simulink model "controlador2"  (R2019a)
settings: Solver=FixedStepDiscrete  StartTime=0.0  StopTime=150  FixedStep=0.1  RelTol=1e-3
undefined symbols (not defined in the file): Angular, Linear
libraries: robotlib x11, fuzblock x1, robotcorelib x1
settings Model: EnablePacing=on  Creator=pizarro  LastModifiedBy=Álvaro Zamorano

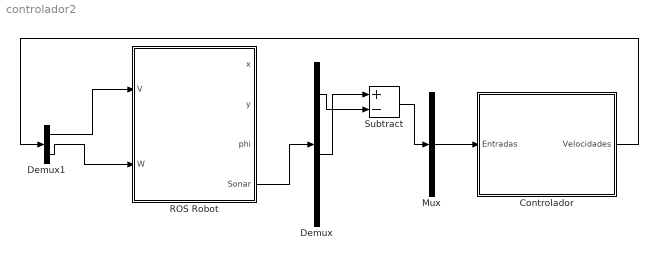
== system controlador2 ==
  Controlador : Subsystem
  Demux : Demux  Outputs=8
  Demux1 : Demux  Outputs=2
  Mux : Mux  Inputs=1
  ROS Robot : Subsystem
  Subtract : Sum  Inputs=+-
  wires:
  ROS Robot/4(Sonar) -> Demux/1
  Mux/1 -> Controlador/1(Entradas)
  Demux1/1 -> ROS Robot/1(V)
  Demux1/2 -> ROS Robot/2(W)
  Controlador/1(Velocidades) -> Demux1/1
  Demux/5 -> Subtract/1
  Subtract/1 -> Mux/1
  Demux/2 -> Subtract/2

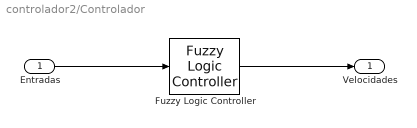
== system controlador2/Controlador ==
  Entradas : Inport
  Fuzzy Logic Controller : fuzblock/Fuzzy Logic  Controller  FIS='Controlador2.fis'  OutputSampleNumber=101  DataType=double  FuzzifiedInputs=off  RuleFiringStrengths=off  RuleOutputs=off  AggregatedOutputs=off  SimulateUsing=Interpreted execution  OutOfRangeInputValueMessage=warning  NoRuleFiredMessage=warning  EmptyOutputFuzzySetMessage=warning
  Velocidades : Outport
  wires:
  Fuzzy Logic Controller/1 -> Velocidades/1
  Entradas/1 -> Fuzzy Logic Controller/1

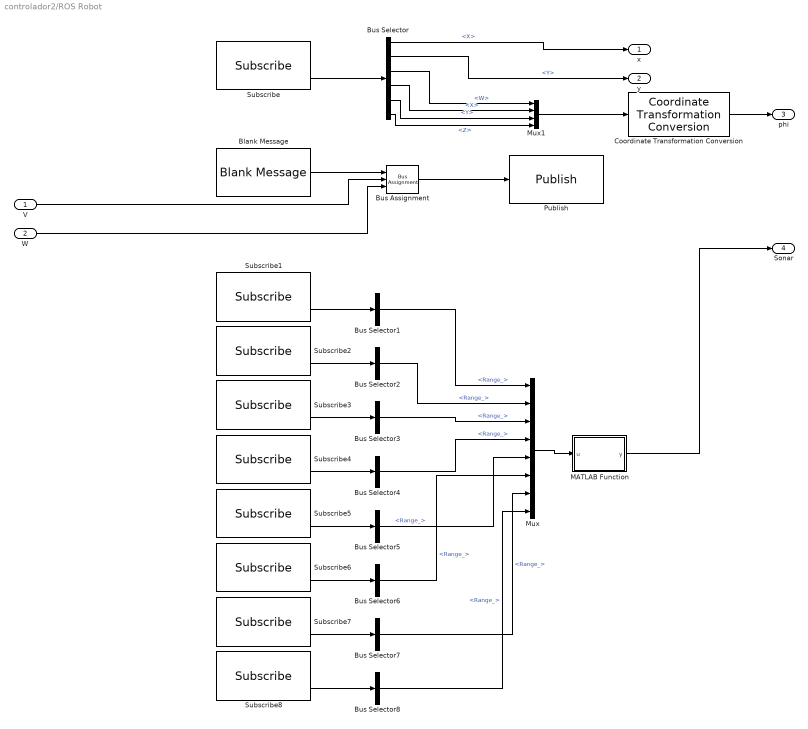
== system controlador2/ROS Robot ==
  V : Inport
  W : Inport  Port=2
  Blank Message : robotlib/Blank Message  messageClass=Message  entityType=geometry_msgs/Twist  messageType=geometry_msgs/Twist  SampleTime=-1
      settings: SourceProductBaseCode=RO
  Bus Assignment : BusAssignment  AssignedSignals=Linear.X,Angular.Z
  Bus Selector : BusSelector  OutputSignals=Pose.Pose.Position.X,Pose.Pose.Position.Y,Pose.Pose.Orientation.W,Pose.Pose.Orientation.X,Pose.Pose.Orientation.Y,Pose.Pose.Orientation.Z
  Bus Selector{1..8} (8 alike) : BusSelector  OutputSignals=Range_
  Coordinate Transformation Conversion : robotcorelib/Coordinate Transformation Conversion  InputRepresentation=Quaternion  InputEulerSequence=ZYX  ShowTrVecInputPort=on  OutputRepresentation=Euler Angles  OutputEulerSequence=ZYX  ShowTrVecOutputPort=on  SimulateUsing=Interpreted execution
      settings: SourceProductBaseCode=RO
  MATLAB Function : MATLAB Function  TreatAsAtomicUnit=on
  Mux : Mux  Inputs=8
  Mux1 : Mux
  Publish : robotlib/Publish  topicSource=Select from ROS network  topic=/robot0/cmd_vel  messageType=geometry_msgs/Twist  messageQueueLength=1
      settings: SourceProductBaseCode=RO
  Subscribe : robotlib/Subscribe  topicSource=Specify your own  topic=/robot0/odom  messageType=nav_msgs/Odometry  sampleTime=-1  messageQueueLength=1
      settings: SourceProductBaseCode=RO
  Subscribe1 : robotlib/Subscribe  topicSource=Select from ROS network  topic=/robot0/sonar_0  messageType=sensor_msgs/Range  sampleTime=-1  messageQueueLength=1
      settings: SourceProductBaseCode=RO
  Subscribe2 : robotlib/Subscribe  topicSource=Select from ROS network  topic=/robot0/sonar_1  messageType=sensor_msgs/Range  sampleTime=-1  messageQueueLength=1
      settings: SourceProductBaseCode=RO
  Subscribe3 : robotlib/Subscribe  topicSource=Select from ROS network  topic=/robot0/sonar_2  messageType=sensor_msgs/Range  sampleTime=-1  messageQueueLength=1
      settings: SourceProductBaseCode=RO
  Subscribe4 : robotlib/Subscribe  topicSource=Select from ROS network  topic=/robot0/sonar_3  messageType=sensor_msgs/Range  sampleTime=-1  messageQueueLength=1
      settings: SourceProductBaseCode=RO
  Subscribe5 : robotlib/Subscribe  topicSource=Select from ROS network  topic=/robot0/sonar_4  messageType=sensor_msgs/Range  sampleTime=-1  messageQueueLength=1
      settings: SourceProductBaseCode=RO
  Subscribe6 : robotlib/Subscribe  topicSource=Select from ROS network  topic=/robot0/sonar_5  messageType=sensor_msgs/Range  sampleTime=-1  messageQueueLength=1
      settings: SourceProductBaseCode=RO
  Subscribe7 : robotlib/Subscribe  topicSource=Select from ROS network  topic=/robot0/sonar_6  messageType=sensor_msgs/Range  sampleTime=-1  messageQueueLength=1
      settings: SourceProductBaseCode=RO
  Subscribe8 : robotlib/Subscribe  topicSource=Select from ROS network  topic=/robot0/sonar_7  messageType=sensor_msgs/Range  sampleTime=-1  messageQueueLength=1
      settings: SourceProductBaseCode=RO
  x : Outport
  y : Outport  Port=2
  phi : Outport  Port=3
  Sonar : Outport  Port=4
  wires:
  Bus Selector/1 -> x/1  "<X>"
  Blank Message/1 -> Bus Assignment/1
  Subscribe/2 -> Bus Selector/1
  Bus Assignment/1 -> Publish/1
  Bus Selector/2 -> y/1  "<Y>"
  Subscribe1/2 -> Bus Selector1/1
  V/1 -> Bus Assignment/2
  W/1 -> Bus Assignment/3
  Subscribe2/2 -> Bus Selector2/1
  Subscribe3/2 -> Bus Selector3/1
  Subscribe5/2 -> Bus Selector5/1
  Subscribe4/2 -> Bus Selector4/1
  Subscribe6/2 -> Bus Selector6/1
  Subscribe7/2 -> Bus Selector7/1
  Bus Selector1/1 -> Mux/1  "<Range_>"
  Bus Selector2/1 -> Mux/2  "<Range_>"
  Bus Selector3/1 -> Mux/3  "<Range_>"
  Bus Selector4/1 -> Mux/4  "<Range_>"
  Bus Selector5/1 -> Mux/5  "<Range_>"
  Bus Selector6/1 -> Mux/6  "<Range_>"
  Bus Selector7/1 -> Mux/7  "<Range_>"
  Subscribe8/2 -> Bus Selector8/1
  Bus Selector8/1 -> Mux/8  "<Range_>"
  Bus Selector/3 -> Mux1/1  "<W>"
  Bus Selector/4 -> Mux1/2  "<X>"
  Bus Selector/5 -> Mux1/3  "<Y>"
  Bus Selector/6 -> Mux1/4  "<Z>"
  Mux1/1 -> Coordinate Transformation Conversion/1
  Coordinate Transformation Conversion/1 -> phi/1
  Mux/1 -> MATLAB Function/1(u)
  MATLAB Function/1(y) -> Sonar/1

== matlab function controlador2/ROS Robot/MATLAB Function ==
  data: u input; y output
function y = fcn(u)
u(isinf(u))=5.0;
y = u;
